simulink model "Advanced_Solar_Tracker"  (R2026a)
settings: Solver=ode45  StopTime=43200  MaxStep=100
libraries: simulink x1, slpidlib x1

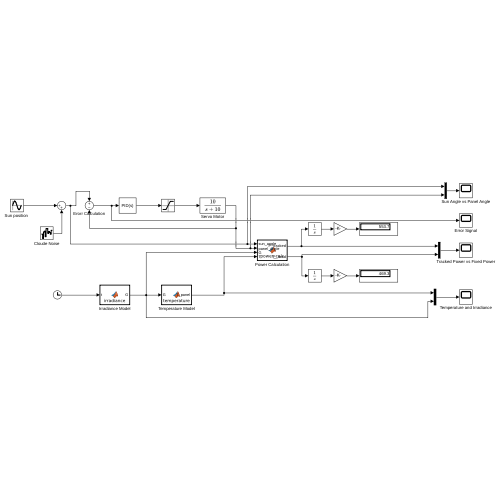
[thumbnail: Simulink's stored preview of the top-level diagram]
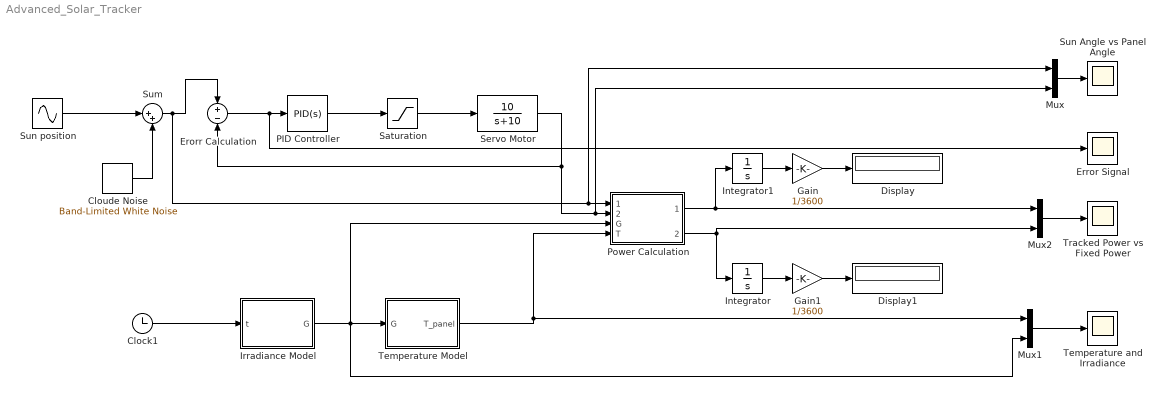
== system Advanced_Solar_Tracker ==
  Clock1 : Clock
  Cloude Noise : simulink/Sources/Band-Limited White Noise  Cov=[0.1]  Ts=0.1  seed=[23341]
  Display : Display
  Display1 : Display
  Erorr Calculation : Sum  Inputs=+-
  Error Signal : Scope
      settings: ActiveDisplayYMinimum=-25.62134163651633  ActiveDisplayYMaximum=22.749393303528297
  Gain : Gain  Gain=1/3600
  Gain1 : Gain  Gain=1/3600
  Integrator : Integrator
  Integrator1 : Integrator
  Irradiance Model : MATLAB Function  TreatAsAtomicUnit=on
  Mux : Mux  Inputs=2
  Mux1 : Mux  Inputs=2
  Mux2 : Mux  Inputs=2
  PID Controller : slpidlib/PID Controller  Controller=PID  Form=Parallel  TimeDomain=Continuous-time  UseExternalTs=off  SampleTime=-1  IntegratorMethod=Forward Euler  FilterMethod=Forward Euler  ControllerParametersSource=internal  P=2  I=0.5  UseKiTs=off  D=0.1  UseExternalDerivativeSource=off  N=100  UseFilter=on  TunerSelectOption=Transfer Function Based (PID Tuner App)  InitialConditionSource=internal  InitialConditionForIntegrator=0  InitialConditionForFilter=0  DifferentiatorICPrevScaledInput=0  ExternalReset=none  TrackingMode=off  Kt=1  LimitOutput=off  SatLimitsSource=internal  UpperSaturationLimit=inf  LowerSaturationLimit=-inf  LinearizeAsGain=on  AntiWindupMode=none  Kb=1  LimitIntegrator=off  UpperIntegratorSaturationLimit=inf  LowerIntegratorSaturationLimit=-inf  POutMin=[]  POutMax=[]  IOutMin=[]  IOutMax=[]  DOutMin=[]  DOutMax=[]  NOutMin=[]  NOutMax=[]  SumOutMin=[]  SumOutMax=[]  SaturationOutMin=[]  SaturationOutMax=[]  PParamMin=[]  PParamMax=[]  IParamMin=[]  IParamMax=[]  DParamMin=[]  DParamMax=[]  NParamMin=[]  NParamMax=[]  KbParamMin=[]  KbParamMax=[]  KtParamMin=[]  KtParamMax=[]  KbOutMin=[]  KbOutMax=[]  KtOutMin=[]  KtOutMax=[]  IntegratorOutMin=[]  IntegratorOutMax=[]  FilterOutMin=[]  FilterOutMax=[]  SumI1OutMin=[]  SumI1OutMax=[]  SumI2OutMin=[]  SumI2OutMax=[]  SumI3OutMin=[]  SumI3OutMax=[]  SumI4OutMin=[]  SumI4OutMax=[]  SumDOutMin=[]  SumDOutMax=[]  DifferentiatorOutMin=[]  DifferentiatorOutMax=[]  FilterDiffOutCoefMin=[]  FilterDiffOutCoefMax=[]  ReciprocalOutMin=[]  ReciprocalOutMax=[]  SumDenOutMin=[]  SumDenOutMax=[]  SumNumOutMin=[]  SumNumOutMax=[]  DivideOutMin=[]  DivideOutMax=[]  UdiffTsProdOutMin=[]  UdiffTsProdOutMax=[]  NTsProdOutMin=[]  NTsProdOutMax=[]  UintegralTsProdOutMin=[]  UintegralTsProdOutMax=[]  UngainTsProdOutMin=[]  UngainTsProdOutMax=[]  ClampingZeroOutDataTypeStr=Inherit: Inherit via back propagation  ClampingZeroOutMin=[]  ClampingZeroOutMax=[]  FilterDenConstantOutDataTypeStr=Inherit: Inherit via back propagation  FilterDenConstantOutMin=[]  FilterDenConstantOutMax=[]  PCopyOutDataTypeStr=Inherit: Inherit via back propagation  PCopyOutMin=[]  PCopyOutMax=[]  NCopyOutDataTypeStr=Inherit: Inherit via back propagation  NCopyOutMin=[]  NCopyOutMax=[]  IntegratorContinuousStateAttributes=''  IntegratorStateMustResolveToSignalObject=off  IntegratorRTWStateStorageClass=Auto  FilterContinuousStateAttributes=''  FilterStateMustResolveToSignalObject=off  FilterRTWStateStorageClass=Auto  ParallelPVariant=InternalParameters  IdealPVariant=Disabled  IVariant=InternalParameters  DVariant=InternalParameters  IntegratorVariant=Continuous  SatVariant=Disabled  AWVariant=Passthrough  PCopyVariant=Disabled  TRVariant=Disabled  FdbkBlocksVariant=Forward  IdealPFdbkVariant=Disabled  SatFdbkVariant=Disabled  DerivativeFilterVariant=ContFilter  NVariant=InternalParameters  NCopyVariant=Disabled  FilterICVariant=InternalICsFilter  IntegratorICVariant=InternalICs  ExternalResetVariant=Disabled  TRSumVariant=Passthrough  SumFdbkVariant=Disabled  SumVariant=Sum_PID  TsampFilterVariant=InternalTs  TsampNgainVariant=Passthrough  TsampIntegralVariant=Disabled_SignalSpec  ExternalSaturationOutDataTypeStr=Inherit: Same as second input  DerivativeSourceVariant=ErrorSignal  PreIntVariant=InternalPreInt
  Power Calculation : MATLAB Function  TreatAsAtomicUnit=on
  Saturation : Saturate  UpperLimit=90  LowerLimit=-90
  Servo Motor : TransferFcn  Numerator=[10]  Denominator=[1 10]
  Sum : Sum  Inputs=|++
  Sun Angle vs Panel Angle : Scope
      settings: ActiveDisplayYMinimum=-343.33189286868384  ActiveDisplayYMaximum=322.70923961598015
  "Sun position " : Sin  Amplitude=90  Frequency=0.000072  SampleTime=0
  Temperature Model : MATLAB Function  TreatAsAtomicUnit=on
  Temperature and Irradiance : Scope
      settings: ActiveDisplayYMinimum=-228.66563628419169  ActiveDisplayYMaximum=1301.8452981608552  DataLoggingVariableName=ScopeData3
  Tracked Power vs Fixed Power : Scope
      settings: ActiveDisplayYMinimum=-8.6328124420373946  ActiveDisplayYMaximum=77.695311978336562  DataLoggingVariableName=ScopeData2
  wires:
  "Sun position "/1 -> Sum/1
  Erorr Calculation/1 -> PID Controller/1, Error Signal/1
  PID Controller/1 -> Saturation/1
  Saturation/1 -> Servo Motor/1
  Servo Motor/1 -> Mux/2, Power Calculation/2(panel_angle), Erorr Calculation/2
  Cloude Noise/1 -> Sum/2
  Clock1/1 -> Irradiance Model/1(t)
  Temperature Model/1(T_panel) -> Power Calculation/4(T), Mux1/1
  Sum/1 -> Erorr Calculation/1, Mux/1, Power Calculation/1(sun_angle)
  Power Calculation/1(P_tracked) -> Mux2/1, Integrator1/1
  Power Calculation/2(P_fixed) -> Integrator/1, Mux2/2
  Gain/1 -> Display/1
  Integrator/1 -> Gain1/1
  Integrator1/1 -> Gain/1
  Gain1/1 -> Display1/1
  Irradiance Model/1(G) -> Power Calculation/3(G), Mux1/2, Temperature Model/1(G)
  Mux/1 -> Sun Angle vs Panel Angle/1
  Mux2/1 -> Tracked Power vs Fixed Power/1
  Mux1/1 -> Temperature and Irradiance/1

== matlab function Advanced_Solar_Tracker/Temperature Model ==
  data: G input; T_panel output
function T_panel = temperature(G)

T_ambient = 25;

T_panel = T_ambient + (G / 800) * 30;

end

== matlab function Advanced_Solar_Tracker/Irradiance Model ==
  data: t input; G output
function G = irradiance(t)

T = 43200;

G = 1000 * sin(pi * t / T);

G = max(0, G);

end

== matlab function Advanced_Solar_Tracker/Power Calculation ==
  data: sun_angle input; P_tracked output; panel_angle input; G input; T input; P_fixed output
function [P_tracked, P_fixed] = power_calc(...
sun_angle, panel_angle, G, T)

Pmax = 100;
eta  = 0.85;

temp_factor = 1 - 0.005 * (T - 25);

error_rad = abs(sun_angle - panel_angle) * pi/180;

P_tracked = Pmax * (G/1000) ...
* eta * temp_factor * cos(error_rad);

P_tracked = max(0, P_tracked);

fixed_error_rad = abs(sun_angle - 45) * pi/180;

P_fixed = Pmax * (G/1000) ...
* eta * temp_factor * cos(fixed_error_rad);

P_fixed = max(0, P_fixed);

end
